simulink model "GuidanceSimV2"  (R2024b)
settings: Solver=FixedStepAuto  StartTime=0.0  StopTime=inf  RelTol=1e-3
values from neighbouring files (symbols this model uses):
  a_max = 10    [GuidanceSimParams.m]
  a_min = -10    [GuidanceSimParams.m]
  gM = asin(2/3*sin(gT-LOS))+LOS    [GuidanceSimParams.m]
  N = 3.5    [GuidanceSimParams.m]
  Rlethal = 1    [GuidanceSimParams.m]
  RM = [xM;zM]    [GuidanceSimParams.m]
  RT = [xT;zT]    [GuidanceSimParams.m]
  Vcinit = MS*cos(gM-LOS)-TS*cos(gT-LOS)    [GuidanceSimParams.m]
  VM = [600*cos(gM),-600*sin(gM)]    [GuidanceSimParams.m]
  VT = [400*cos(gT),-400*sin(gT)]    [GuidanceSimParams.m]
  Wn_hom = 7    [GuidanceSimParams.m]
undefined symbols (not defined in the file or in its folder): drawMissile
libraries: simulink x2, simulink_extras x2, aerolibanim x1
settings Model: Creator=Ameya  LastModifiedBy=Ameya

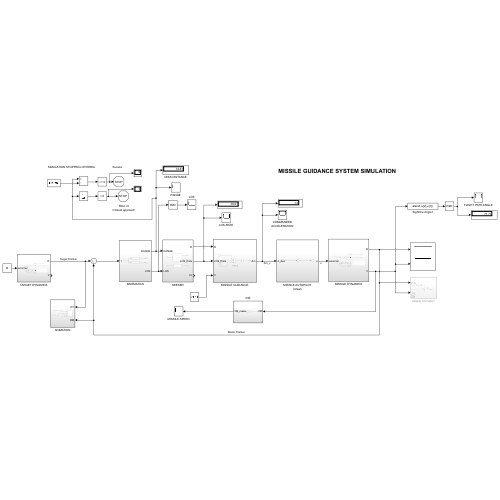
[thumbnail: Simulink's stored preview of the top-level diagram]
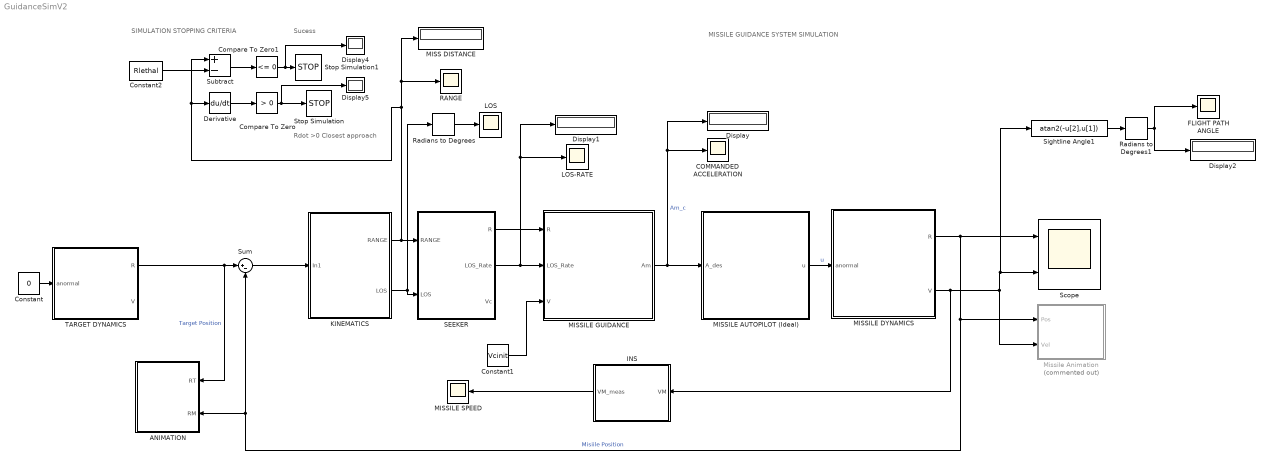
== system GuidanceSimV2 ==
  note: MISSILE GUIDANCE SYSTEM SIMULATION
  note: Rdot >0
      | Closest approach
  note: SIMULATION STOPPING CRITERIA
  note: Sucess
  ANIMATION : Subsystem
  COMMANDED ACCELERATION : Scope
  Compare To Zero : simulink/Logic and Bit Operations/Compare To Zero  relop=>  OutDataTypeStr=boolean
  Compare To Zero1 : simulink/Logic and Bit Operations/Compare To Zero  relop=<=  OutDataTypeStr=boolean
  Constant : Constant  Value=0
  Constant1 : Constant  Value=Vcinit
  Constant2 : Constant  Value=Rlethal
  Derivative : Derivative
  Display{,1..2,4..5} (5 alike) : Display
  FLIGHT PATH ANGLE : Scope
  INS : Subsystem
  KINEMATICS : Subsystem
  LOS : Scope
  LOS-RATE : Scope
  MISS DISTANCE : Display
  MISSILE AUTOPILOT (Ideal) : Subsystem
  MISSILE DYNAMICS : Subsystem
  MISSILE GUIDANCE : Subsystem
  MISSILE SPEED : Scope
  Missile Animation : Subsystem  Commented=on
  RANGE : Scope
  Radians to Degrees : simulink_extras/Transformations/Radians to Degrees
  Radians to Degrees1 : simulink_extras/Transformations/Radians to Degrees
  SEEKER : Subsystem
  Scope : Scope  NumInputPorts=2
  Sightline Angle1 : Fcn  Expr=atan2(-u[2],u[1])
  Stop Simulation : Stop
  Stop Simulation1 : Stop
  Subtract : Sum  Inputs=+-
  Sum : Sum  Inputs=|+-
  TARGET DYNAMICS : Subsystem
  wires:
  MISSILE GUIDANCE/1(Am) -> COMMANDED ACCELERATION/1, Display/1, MISSILE AUTOPILOT (Ideal)/1(A_des)  "Am_c"
  Constant/1 -> TARGET DYNAMICS/1(anormal)
  Radians to Degrees/1 -> LOS/1
  Compare To Zero/1 -> Display5/1, Stop Simulation/1
  Derivative/1 -> Compare To Zero/1
  Constant2/1 -> Subtract/2
  Subtract/1 -> Compare To Zero1/1
  Compare To Zero1/1 -> Display4/1, Stop Simulation1/1
  INS/1(VM_meas) -> MISSILE SPEED/1
  TARGET DYNAMICS/1(R) -> ANIMATION/1(RT), Sum/1  "Target Position"
  MISSILE DYNAMICS/1(R) -> ANIMATION/2(RM), Sum/2, Missile Animation/1(Pos), Scope/1  "Misiile Position"
  Sum/1 -> KINEMATICS/1(In1)
  KINEMATICS/1(RANGE) -> Derivative/1, Subtract/1, RANGE/1, MISS DISTANCE/1, SEEKER/1(RANGE)
  KINEMATICS/2(LOS) -> Radians to Degrees/1, SEEKER/2(LOS)
  SEEKER/2(LOS_Rate) -> Display1/1, LOS-RATE/1, MISSILE GUIDANCE/2(LOS_Rate)
  SEEKER/1(R) -> MISSILE GUIDANCE/1(R)
  MISSILE AUTOPILOT (Ideal)/1(u) -> MISSILE DYNAMICS/1(anormal)  "u"
  MISSILE DYNAMICS/2(V) -> INS/1(VM), Sightline Angle1/1, Scope/2, Missile Animation/2(Vel)
  Sightline Angle1/1 -> Radians to Degrees1/1
  Radians to Degrees1/1 -> FLIGHT PATH ANGLE/1, Display2/1
  Constant1/1 -> MISSILE GUIDANCE/3(V)

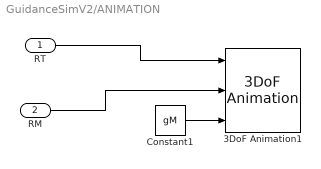
== system GuidanceSimV2/ANIMATION ==
  RT : Inport
  RM : Inport  Port=2
  3DoF Animation1 : aerolibanim/3DoF Animation  u1=[0 5000 -2000 2000 -5050 -3]  u2=0.05  u3=1  u5=Fly alongside  u6=[2000 500 -3150]  u7=10  u8=on
  Constant1 : Constant  Value=gM
  wires:
  Constant1/1 -> 3DoF Animation1/3
  RT/1 -> 3DoF Animation1/1
  RM/1 -> 3DoF Animation1/2

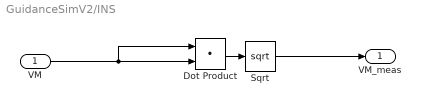
== system GuidanceSimV2/INS ==
  VM : Inport
  Dot Product : DotProduct  OutDataTypeStr=Inherit: Inherit via internal rule
  Sqrt : Sqrt
  VM_meas : Outport
  wires:
  Dot Product/1 -> Sqrt/1
  Sqrt/1 -> VM_meas/1
  VM/1 -> Dot Product/1, Dot Product/2

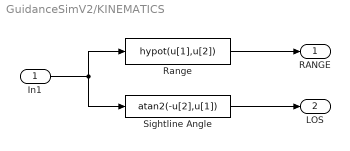
== system GuidanceSimV2/KINEMATICS ==
  In1 : Inport
  Range : Fcn  Expr=hypot(u[1],u[2])
  Sightline Angle : Fcn  Expr=atan2(-u[2],u[1])
  RANGE : Outport
  LOS : Outport  Port=2
  wires:
  In1/1 -> Range/1, Sightline Angle/1
  Range/1 -> RANGE/1
  Sightline Angle/1 -> LOS/1

== system GuidanceSimV2/MISSILE AUTOPILOT (Ideal) ==
  A_des : Inport
  Gain : Gain
  u : Outport
  wires:
  A_des/1 -> Gain/1
  Gain/1 -> u/1

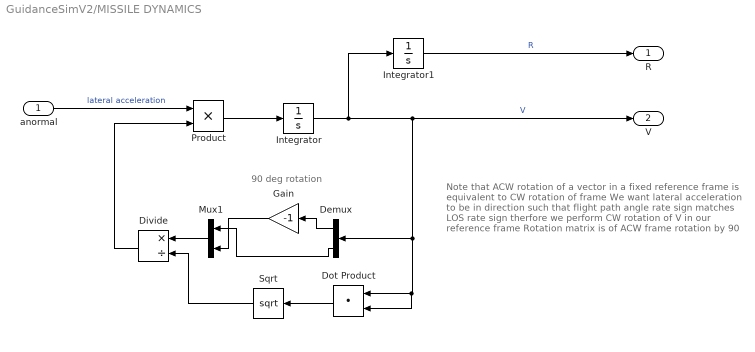
== system GuidanceSimV2/MISSILE DYNAMICS ==
  note: 90 deg rotation
  note: Note that ACW rotation of a vector in
      | a fixed reference frame is equivalent to
      | CW rotation of frame
      |
      | We want lateral acceleration to be in direction
      | such that flight path angle rate sign matches LOS rate sign
      | therfore we perform CW rotation of V in our reference frame
      | Rotation matrix is of ACW frame rotation by 90
  anormal : Inport
  Demux : Demux  Outputs=2
  Divide : Product  Inputs=*/
  Dot Product : DotProduct  OutDataTypeStr=Inherit: Inherit via internal rule
  Gain : Gain  Gain=-1
  Integrator : Integrator  InitialCondition=VM
  Integrator1 : Integrator  InitialCondition=RM
  Mux1 : Mux  Inputs=2
  Product : Product
  Sqrt : Sqrt
  R : Outport
  V : Outport  Port=2
  wires:
  anormal/1 -> Product/1  "lateral acceleration"
  Integrator1/1 -> R/1  "R"
  Demux/2 -> Mux1/1
  Dot Product/1 -> Sqrt/1
  Demux/1 -> Gain/1
  Sqrt/1 -> Divide/2
  Divide/1 -> Product/2
  Mux1/1 -> Divide/1
  Gain/1 -> Mux1/2
  Product/1 -> Integrator/1
  Integrator/1 -> Integrator1/1, V/1, Dot Product/2, Dot Product/1, Demux/1  "V"

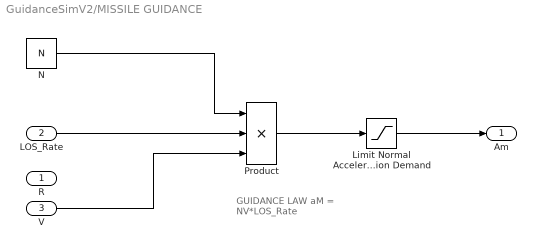
== system GuidanceSimV2/MISSILE GUIDANCE ==
  note: GUIDANCE LAW
      | aM = NV*LOS_Rate
  R : Inport
  LOS_Rate : Inport  Port=2
  V : Inport  Port=3
  Limit Normal Acceleration Demand : Saturate  UpperLimit=a_max+100  LowerLimit=a_min
  N : Constant  Value=N
  Product : Product  Inputs=3
  Am : Outport
  wires:
  N/1 -> Product/1
  Product/1 -> Limit Normal Acceleration Demand/1
  LOS_Rate/1 -> Product/2
  V/1 -> Product/3
  Limit Normal Acceleration Demand/1 -> Am/1

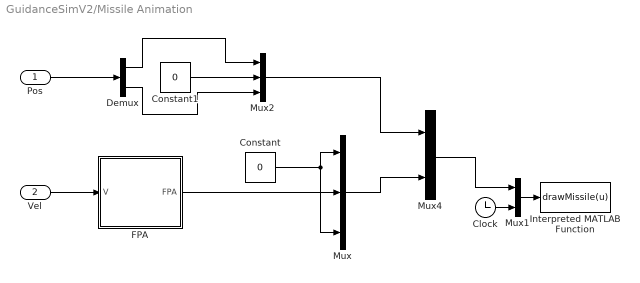
== system GuidanceSimV2/Missile Animation ==
  Pos : Inport
  Vel : Inport  Port=2
  Clock : Clock
  Constant : Constant  Value=0
  Constant1 : Constant  Value=0
  Demux : Demux  Outputs=2
  FPA : Subsystem
  Interpreted MATLAB Function : MATLABFcn  MATLABFcn=drawMissile(u)  OutputDimensions=0
  Mux : Mux  Inputs=3
  Mux1 : Mux  Inputs=2
  Mux2 : Mux  Inputs=3
  Mux4 : Mux  Inputs=2
  wires:
  Clock/1 -> Mux1/2
  Mux1/1 -> Interpreted MATLAB Function/1
  Constant/1 -> Mux/3, Mux/1
  Pos/1 -> Demux/1
  Constant1/1 -> Mux2/2
  Demux/1 -> Mux2/1
  Demux/2 -> Mux2/3
  Vel/1 -> FPA/1(V)
  Mux4/1 -> Mux1/1
  Mux2/1 -> Mux4/1
  Mux/1 -> Mux4/2
  FPA/1(FPA) -> Mux/2

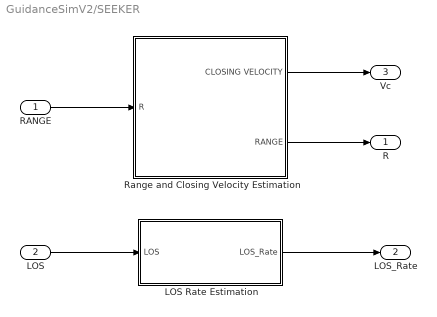
== system GuidanceSimV2/SEEKER ==
  RANGE : Inport
  LOS : Inport  Port=2
  LOS Rate Estimation : Subsystem
  Range and Closing Velocity Estimation : Subsystem
  R : Outport  InitialOutput=0  VectorParamsAs1DForOutWhenUnconnected=off
  LOS_Rate : Outport  Port=2
  Vc : Outport  Port=3  InitialOutput=0  VectorParamsAs1DForOutWhenUnconnected=off
  wires:
  RANGE/1 -> Range and Closing Velocity Estimation/1(R)
  Range and Closing Velocity Estimation/1(CLOSING VELOCITY) -> Vc/1
  Range and Closing Velocity Estimation/2(RANGE) -> R/1
  LOS/1 -> LOS Rate Estimation/1(LOS)
  LOS Rate Estimation/1(LOS_Rate) -> LOS_Rate/1

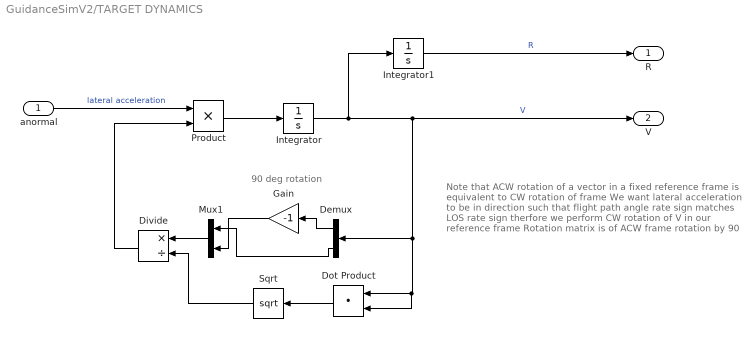
== system GuidanceSimV2/TARGET DYNAMICS ==
  note: 90 deg rotation
  note: Note that ACW rotation of a vector in
      | a fixed reference frame is equivalent to
      | CW rotation of frame
      |
      | We want lateral acceleration to be in direction
      | such that flight path angle rate sign matches LOS rate sign
      | therfore we perform CW rotation of V in our reference frame
      | Rotation matrix is of ACW frame rotation by 90
  anormal : Inport
  Demux : Demux  Outputs=2
  Divide : Product  Inputs=*/
  Dot Product : DotProduct  OutDataTypeStr=Inherit: Inherit via internal rule
  Gain : Gain  Gain=-1
  Integrator : Integrator  InitialCondition=VT
  Integrator1 : Integrator  InitialCondition=RT
  Mux1 : Mux  Inputs=2
  Product : Product
  Sqrt : Sqrt
  R : Outport
  V : Outport  Port=2
  wires:
  anormal/1 -> Product/1  "lateral acceleration"
  Integrator1/1 -> R/1  "R"
  Demux/2 -> Mux1/1
  Dot Product/1 -> Sqrt/1
  Demux/1 -> Gain/1
  Sqrt/1 -> Divide/2
  Divide/1 -> Product/2
  Mux1/1 -> Divide/1
  Gain/1 -> Mux1/2
  Product/1 -> Integrator/1
  Integrator/1 -> Integrator1/1, V/1, Dot Product/2, Dot Product/1, Demux/1  "V"

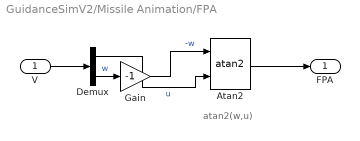
== system GuidanceSimV2/Missile Animation/FPA ==
  note: atan2(w,u)
  V : Inport
  Atan2 : Trigonometry  Operator=atan2
  Demux : Demux  Outputs=2
  Gain : Gain  Gain=-1
  FPA : Outport
  wires:
  V/1 -> Demux/1
  Demux/2 -> Gain/1  "w"
  Demux/1 -> Atan2/2  "u"
  Atan2/1 -> FPA/1
  Gain/1 -> Atan2/1  "-w"

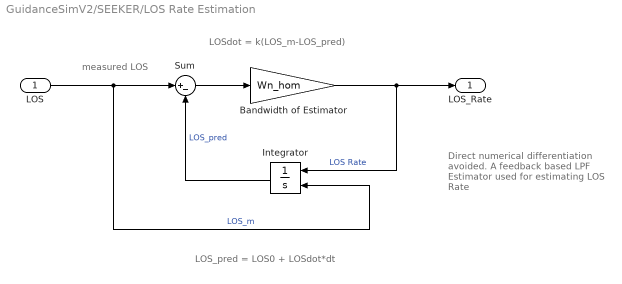
== system GuidanceSimV2/SEEKER/LOS Rate Estimation ==
  note: LOS_pred = LOS0 + LOSdot*dt
  note: LOSdot = k(LOS_m-LOS_pred)
  note: measured LOS
  note: Direct numerical differentiation avoided.
      | A feedback based LPF Estimator used for estimating LOS Rate
  LOS : Inport
  Bandwidth of Estimator : Gain  Gain=Wn_hom  SaturateOnIntegerOverflow=on  OutDataTypeStr=Inherit: Same as input  ParamDataTypeStr=Inherit: Same as input
  Integrator : Integrator  InitialConditionSource=external
  Sum : Sum  Inputs=|+-
  LOS_Rate : Outport
  wires:
  LOS/1 -> Sum/1, Integrator/2  "LOS_m"
  Sum/1 -> Bandwidth of Estimator/1
  Bandwidth of Estimator/1 -> Integrator/1, LOS_Rate/1  "LOS Rate"
  Integrator/1 -> Sum/2  "LOS_pred"

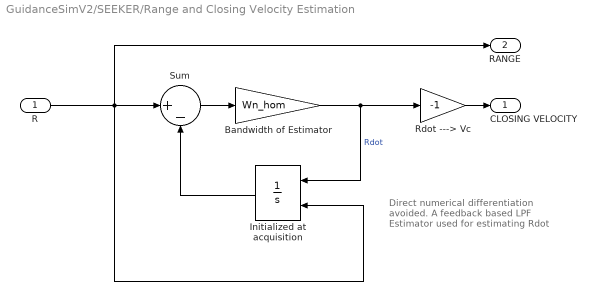
== system GuidanceSimV2/SEEKER/Range and Closing Velocity Estimation ==
  note: Direct numerical differentiation avoided.
      | A feedback based LPF Estimator used for estimating Rdot
  R : Inport
  Bandwidth of Estimator : Gain  Gain=Wn_hom  SaturateOnIntegerOverflow=on  OutDataTypeStr=Inherit: Same as input  ParamDataTypeStr=Inherit: Same as input
  Initialized at acquisition : Integrator  InitialConditionSource=external
  Rdot ---> Vc : Gain  Gain=-1  SaturateOnIntegerOverflow=on  OutDataTypeStr=Inherit: Same as input  ParamDataTypeStr=Inherit: Same as input
  Sum : Sum  Inputs=|+-  InputSameDT=on  SaturateOnIntegerOverflow=on  OutDataTypeStr=Inherit: Same as first input
  CLOSING VELOCITY : Outport  InitialOutput=0  VectorParamsAs1DForOutWhenUnconnected=off
  RANGE : Outport  Port=2  InitialOutput=0  VectorParamsAs1DForOutWhenUnconnected=off
  wires:
  R/1 -> Sum/1, Initialized at acquisition/2, RANGE/1
  Initialized at acquisition/1 -> Sum/2
  Bandwidth of Estimator/1 -> Rdot ---> Vc/1, Initialized at acquisition/1  "Rdot"
  Rdot ---> Vc/1 -> CLOSING VELOCITY/1
  Sum/1 -> Bandwidth of Estimator/1
